simulink subsystem "FOC_Sub_StateMch"  (R2020b)
settings: Solver=VariableStepAuto  StartTime=0.0  StopTime=10.0  RelTol=1e-3
undefined symbols (not defined in the file or in its folder): innerPI, outerPI, Tctr
libraries: mcbcontrolslib x3
settings Model: Creator=k  LastModifiedBy=wangdi
settings OptimizationCC: DefaultParameterBehavior=Inlined  EnhancedBackFolding=on  PassReuseOutputArgsAs=Individual arguments  ZeroExternalMemoryAtStartup=off  ZeroInternalMemoryAtStartup=off  OptimizeBlockOrder=speed  DifferentSizesBufferReuse=on  OptimizationCustomize=off  EfficientTunableParamExpr=on
settings DebuggingCC: ParameterTunabilityLossMsg=error
settings SFSimCC: MATLABDynamicMemAlloc=off
settings RTWCC: Description=Embedded Coder  SystemTargetFile=ert.tlc  TemplateMakefile=ert_default_tmf
settings CodeAppCC: ForceParamTrailComments=on  IgnoreCustomStorageClasses=off  OperatorAnnotations=on  SimulinkDataObjDesc=on  SFDataObjDesc=on  InsertBlockDesc=on
settings ERTTargetCC: TargetLangStandard=C99 (ISO)  GenerateSampleERTMain=on  InlinedParameterPlacement=NonHierarchical  ERTCustomFileTemplate=example_file_process.tlc

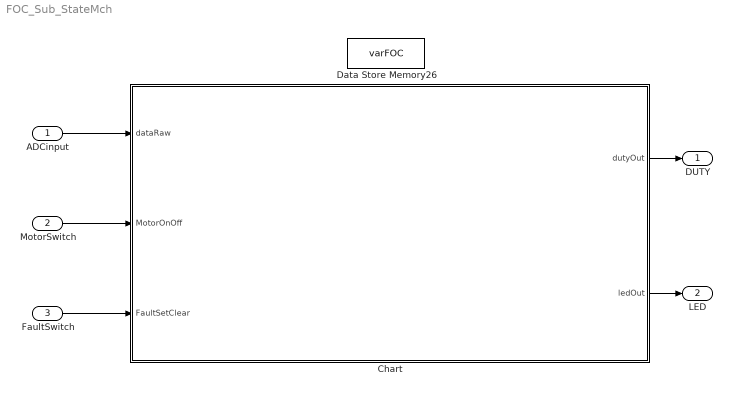
== system FOC_Sub_StateMch ==
  ADCinput : Inport  OutDataTypeStr=uint16  PortDimensions=5
  MotorSwitch : Inport  Port=2  OutDataTypeStr=boolean  PortDimensions=1
  FaultSwitch : Inport  Port=3  OutDataTypeStr=boolean  PortDimensions=1
  Chart : Stateflow chart  TreatAsAtomicUnit=on
  Data Store Memory26 : DataStoreMemory  DataStoreName=varFOC  ReadBeforeWriteMsg=warning  WriteAfterWriteMsg=warning  WriteAfterReadMsg=warning  ShowAdditionalParam=off  OutDataTypeStr=Bus: structFOC
  DUTY : Outport  PortDimensions=3
  LED : Outport  Port=2  PortDimensions=3
  wires:
  Chart/1(dutyOut) -> DUTY/1
  FaultSwitch/1 -> Chart/3(FaultSetClear)
  MotorSwitch/1 -> Chart/2(MotorOnOff)
  ADCinput/1 -> Chart/1(dataRaw)
  Chart/2(ledOut) -> LED/1

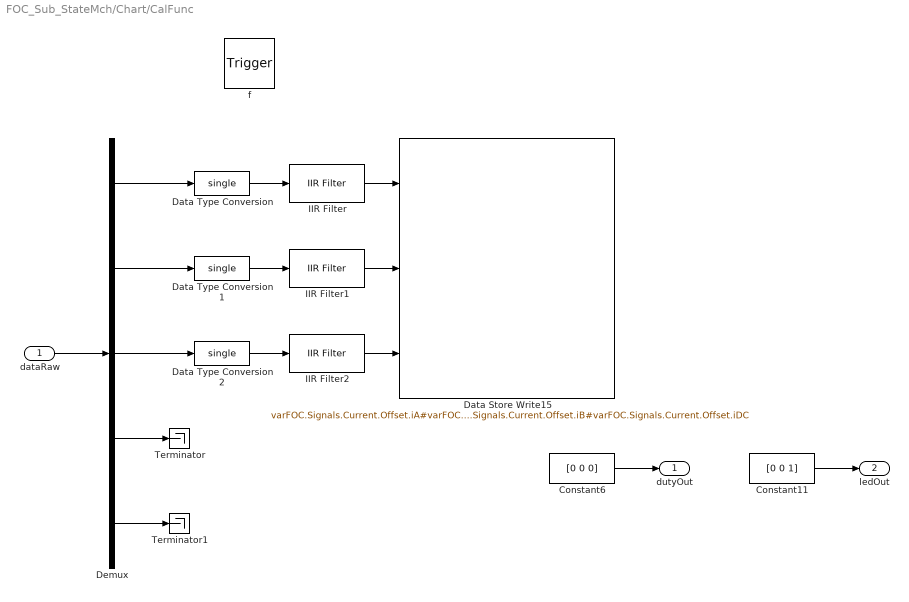
== system FOC_Sub_StateMch/Chart/CalFunc ==
  dataRaw : Inport  OutDataTypeStr=uint16  PortDimensions=5
  f : TriggerPort  TriggerType=function-call  VariantControl=(inherit)
      settings: CopyFcn=Stateflow.SLINSF.SimulinkMan.removeBlockPreDeleteFcn  PreDeleteFcn=Stateflow.SLINSF.SimulinkMan.unsafePredeleteFcn
  Constant11 : Constant  Value=[0 0 1]  OutDataTypeStr=boolean
  Constant6 : Constant  Value=[0 0 0]  OutDataTypeStr=single
  Data Store Write15 : DataStoreWrite  DataStoreName=varFOC  DataStoreElements=varFOC.Signals.Current.Offset.iA#varFOC.Signals.Current.Offset.iB#varFOC.Signals.Current.Offset.iDC
  Data Type Conversion : DataTypeConversion  OutDataTypeStr=single
  Data Type Conversion1 : DataTypeConversion  OutDataTypeStr=single
  Data Type Conversion2 : DataTypeConversion  OutDataTypeStr=single
  Demux : Demux  Outputs=5
  IIR Filter : mcbcontrolslib/IIR Filter  Filter_constant=0.001
      settings: SourceProductBaseCode=MT
  IIR Filter1 : mcbcontrolslib/IIR Filter  Filter_constant=0.001
      settings: SourceProductBaseCode=MT
  IIR Filter2 : mcbcontrolslib/IIR Filter  Filter_constant=0.001
      settings: SourceProductBaseCode=MT
  Terminator : Terminator
  Terminator1 : Terminator
  dutyOut : Outport  OutDataTypeStr=single
  ledOut : Outport  Port=2
  wires:
  IIR Filter2/1 -> Data Store Write15/3
  IIR Filter1/1 -> Data Store Write15/2
  Data Type Conversion2/1 -> IIR Filter2/1
  Demux/3 -> Data Type Conversion2/1
  Data Type Conversion1/1 -> IIR Filter1/1
  IIR Filter/1 -> Data Store Write15/1
  Demux/2 -> Data Type Conversion1/1
  Demux/1 -> Data Type Conversion/1
  Data Type Conversion/1 -> IIR Filter/1
  Demux/4 -> Terminator/1
  Demux/5 -> Terminator1/1
  dataRaw/1 -> Demux/1
  Constant6/1 -> dutyOut/1
  Constant11/1 -> ledOut/1

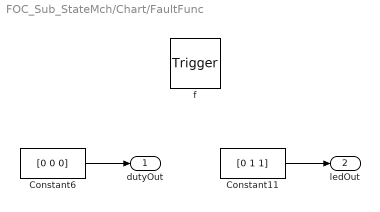
== system FOC_Sub_StateMch/Chart/FaultFunc ==
  f : TriggerPort  TriggerType=function-call  VariantControl=(inherit)
      settings: CopyFcn=Stateflow.SLINSF.SimulinkMan.removeBlockPreDeleteFcn  PreDeleteFcn=Stateflow.SLINSF.SimulinkMan.unsafePredeleteFcn
  Constant11 : Constant  Value=[0 1 1]  OutDataTypeStr=boolean
  Constant6 : Constant  Value=[0 0 0]  OutDataTypeStr=single
  dutyOut : Outport  OutDataTypeStr=single
  ledOut : Outport  Port=2
  wires:
  Constant6/1 -> dutyOut/1
  Constant11/1 -> ledOut/1

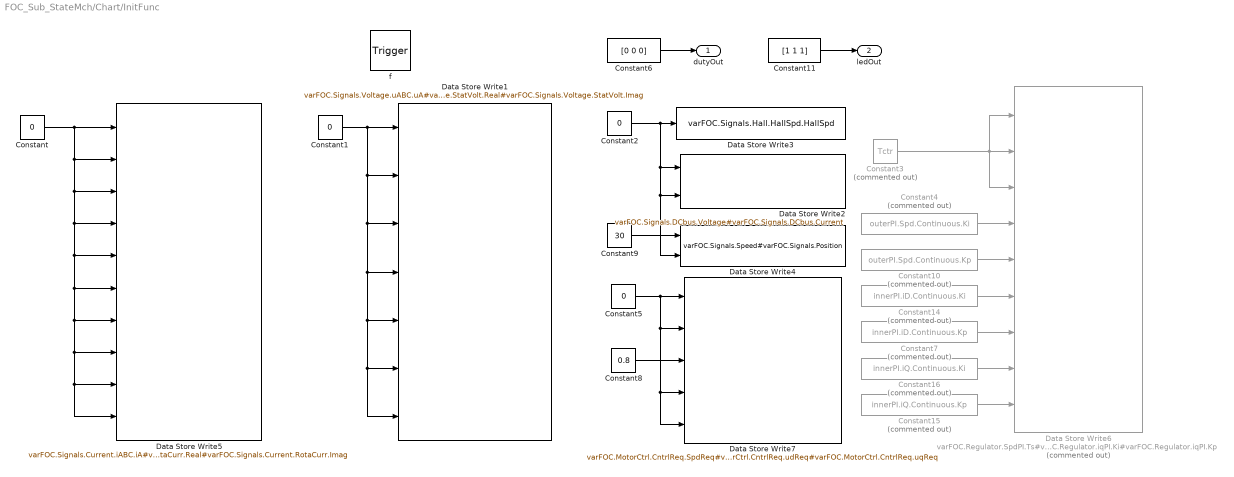
== system FOC_Sub_StateMch/Chart/InitFunc ==
  f : TriggerPort  TriggerType=function-call  VariantControl=(inherit)
      settings: CopyFcn=Stateflow.SLINSF.SimulinkMan.removeBlockPreDeleteFcn  PreDeleteFcn=Stateflow.SLINSF.SimulinkMan.unsafePredeleteFcn
  Constant{,1..2,5} (4 alike) : Constant  Value=0  OutDataTypeStr=single
  Constant10 : Constant  Commented=on  Value=outerPI.Spd.Continuous.Kp  OutDataTypeStr=single
  Constant11 : Constant  Value=[1 1 1]  OutDataTypeStr=boolean
  Constant14 : Constant  Commented=on  Value=innerPI.iD.Continuous.Ki  OutDataTypeStr=single
  Constant15 : Constant  Commented=on  Value=innerPI.iQ.Continuous.Kp  OutDataTypeStr=single
  Constant16 : Constant  Commented=on  Value=innerPI.iQ.Continuous.Ki  OutDataTypeStr=single
  Constant3 : Constant  Commented=on  Value=Tctr  OutDataTypeStr=single
  Constant4 : Constant  Commented=on  Value=outerPI.Spd.Continuous.Ki  OutDataTypeStr=single
  Constant6 : Constant  Value=[0 0 0]  OutDataTypeStr=single
  Constant7 : Constant  Commented=on  Value=innerPI.iD.Continuous.Kp  OutDataTypeStr=single
  Constant8 : Constant  Value=0.8  OutDataTypeStr=single
  Constant9 : Constant  Value=30  OutDataTypeStr=single
  Data Store Write1 : DataStoreWrite  DataStoreName=varFOC  DataStoreElements=varFOC.Signals.Voltage.uABC.uA#varFOC.Signals.Voltage.uABC.uB#varFOC.Signals.Voltage.uABC.uC#varFOC.Signals.Voltage.RotaVolt.Real#varFOC.Signals.Voltage.RotaVolt.Imag#varFOC.Signals.Voltage.StatVolt.Real#varFOC.Signals.Voltage.StatVolt.Imag
  Data Store Write2 : DataStoreWrite  DataStoreName=varFOC  DataStoreElements=varFOC.Signals.DCbus.Voltage#varFOC.Signals.DCbus.Current
  Data Store Write3 : DataStoreWrite  DataStoreName=varFOC  DataStoreElements=varFOC.Signals.Hall.HallSpd.HallSpd
  Data Store Write4 : DataStoreWrite  DataStoreName=varFOC  DataStoreElements=varFOC.Signals.Speed#varFOC.Signals.Position
  Data Store Write5 : DataStoreWrite  DataStoreName=varFOC  DataStoreElements=varFOC.Signals.Current.iABC.iA#varFOC.Signals.Current.iABC.iB#varFOC.Signals.Current.iABC.iC#varFOC.Signals.Current.Offset.iA#varFOC.Signals.Current.Offset.iB#varFOC.Signals.Current.Offset.iDC#varFOC.Signals.Current.StatCurr.Real#varFOC.Signals.Current.StatCurr.Imag#varFOC.Signals.Current.RotaCurr.Real#varFOC.Signals.Current.RotaCurr.Imag
  Data Store Write6 : DataStoreWrite  Commented=on  DataStoreName=varFOC  DataStoreElements=varFOC.Regulator.SpdPI.Ts#varFOC.Regulator.idPI.Ts#varFOC.Regulator.iqPI.Ts#varFOC.Regulator.SpdPI.Ki#varFOC.Regulator.SpdPI.Kp#varFOC.Regulator.idPI.Ki#varFOC.Regulator.idPI.Kp#varFOC.Regulator.iqPI.Ki#varFOC.Regulator.iqPI.Kp
  Data Store Write7 : DataStoreWrite  DataStoreName=varFOC  DataStoreElements=varFOC.MotorCtrl.CntrlReq.SpdReq#varFOC.MotorCtrl.CntrlReq.idReq#varFOC.MotorCtrl.CntrlReq.iqReq#varFOC.MotorCtrl.CntrlReq.udReq#varFOC.MotorCtrl.CntrlReq.uqReq
  dutyOut : Outport  OutDataTypeStr=single
  ledOut : Outport  Port=2
  wires:
  Constant4/1 -> Data Store Write6/4
  Constant10/1 -> Data Store Write6/5
  Constant16/1 -> Data Store Write6/8
  Constant/1 -> Data Store Write5/1, Data Store Write5/9, Data Store Write5/10, Data Store Write5/8, Data Store Write5/7, Data Store Write5/6, Data Store Write5/5, Data Store Write5/4, Data Store Write5/3, Data Store Write5/2
  Constant9/1 -> Data Store Write4/1
  Constant8/1 -> Data Store Write7/3
  Constant14/1 -> Data Store Write6/6
  Constant5/1 -> Data Store Write7/5, Data Store Write7/4, Data Store Write7/2, Data Store Write7/1
  Constant7/1 -> Data Store Write6/7
  Constant2/1 -> Data Store Write4/2, Data Store Write2/2, Data Store Write2/1, Data Store Write3/1
  Constant15/1 -> Data Store Write6/9
  Constant3/1 -> Data Store Write6/1, Data Store Write6/3, Data Store Write6/2
  Constant1/1 -> Data Store Write1/7, Data Store Write1/6, Data Store Write1/5, Data Store Write1/4, Data Store Write1/3, Data Store Write1/2, Data Store Write1/1
  Constant6/1 -> dutyOut/1
  Constant11/1 -> ledOut/1

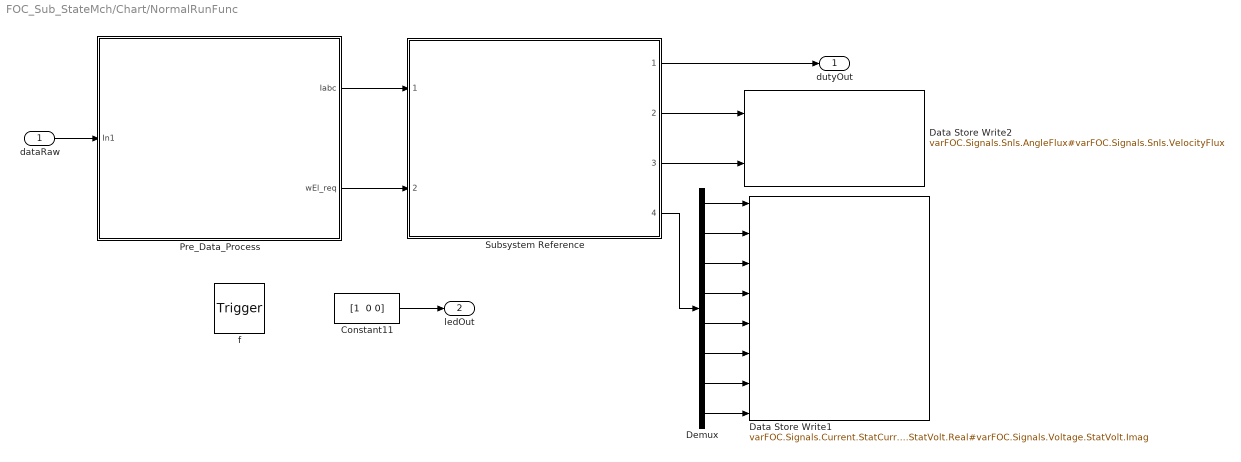
== system FOC_Sub_StateMch/Chart/NormalRunFunc ==
  dataRaw : Inport  OutDataTypeStr=uint16  PortDimensions=5
  f : TriggerPort  TriggerType=function-call  VariantControl=(inherit)
      settings: CopyFcn=Stateflow.SLINSF.SimulinkMan.removeBlockPreDeleteFcn  PreDeleteFcn=Stateflow.SLINSF.SimulinkMan.unsafePredeleteFcn
  Constant11 : Constant  Value="[1  0 0]"  OutDataTypeStr=boolean
  Data Store Write1 : DataStoreWrite  DataStoreName=varFOC  DataStoreElements=varFOC.Signals.Current.StatCurr.Real#varFOC.Signals.Current.StatCurr.Imag#varFOC.Signals.Current.RotaCurr.Real#varFOC.Signals.Current.RotaCurr.Imag#varFOC.Signals.Voltage.RotaVolt.Real#varFOC.Signals.Voltage.RotaVolt.Imag#varFOC.Signals.Voltage.StatVolt.Real#varFOC.Signals.Voltage.StatVolt.Imag
  Data Store Write2 : DataStoreWrite  DataStoreName=varFOC  DataStoreElements=varFOC.Signals.Snls.AngleFlux#varFOC.Signals.Snls.VelocityFlux
  Demux : Demux  Outputs=8
  Pre_Data_Process : Subsystem
  Subsystem Reference : Subsystem  ReferencedSubsystem=FOC_Sub_CoreAlgoithm
  dutyOut : Outport  OutDataTypeStr=single
  ledOut : Outport  Port=2
  wires:
  Pre_Data_Process/2(wEl_req) -> Subsystem Reference/2
  Pre_Data_Process/1(Iabc) -> Subsystem Reference/1
  Subsystem Reference/3 -> Data Store Write2/2
  Subsystem Reference/2 -> Data Store Write2/1
  Subsystem Reference/4 -> Demux/1
  Constant11/1 -> ledOut/1
  Subsystem Reference/1 -> dutyOut/1
  dataRaw/1 -> Pre_Data_Process/1(In1)
  Demux/1 -> Data Store Write1/1
  Demux/2 -> Data Store Write1/2
  Demux/3 -> Data Store Write1/3
  Demux/4 -> Data Store Write1/4
  Demux/5 -> Data Store Write1/5
  Demux/6 -> Data Store Write1/6
  Demux/7 -> Data Store Write1/7
  Demux/8 -> Data Store Write1/8

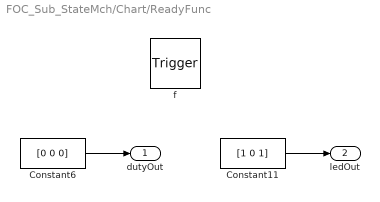
== system FOC_Sub_StateMch/Chart/ReadyFunc ==
  f : TriggerPort  TriggerType=function-call  VariantControl=(inherit)
      settings: CopyFcn=Stateflow.SLINSF.SimulinkMan.removeBlockPreDeleteFcn  PreDeleteFcn=Stateflow.SLINSF.SimulinkMan.unsafePredeleteFcn
  Constant11 : Constant  Value=[1 0 1]  OutDataTypeStr=boolean
  Constant6 : Constant  Value=[0 0 0]  OutDataTypeStr=single
  dutyOut : Outport  OutDataTypeStr=single
  ledOut : Outport  Port=2
  wires:
  Constant11/1 -> ledOut/1
  Constant6/1 -> dutyOut/1

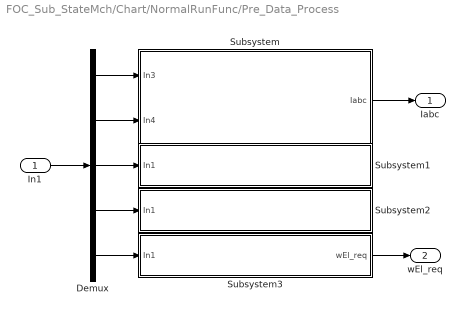
== system FOC_Sub_StateMch/Chart/NormalRunFunc/Pre_Data_Process ==
  In1 : Inport
  Demux : Demux  Outputs=5
  Subsystem : Subsystem
  Subsystem1 : Subsystem
  Subsystem2 : Subsystem
  Subsystem3 : Subsystem
  Iabc : Outport
  wEl_req : Outport  Port=2
  wires:
  Subsystem/1(Iabc) -> Iabc/1
  Demux/4 -> Subsystem2/1(In1)
  Demux/1 -> Subsystem/1(In3)
  Demux/5 -> Subsystem3/1(In1)
  Demux/3 -> Subsystem1/1(In1)
  Demux/2 -> Subsystem/2(In4)
  In1/1 -> Demux/1
  Subsystem3/1(wEl_req) -> wEl_req/1

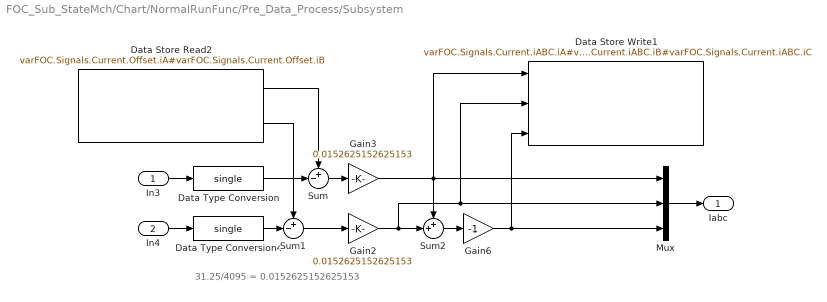
== system FOC_Sub_StateMch/Chart/NormalRunFunc/Pre_Data_Process/Subsystem ==
  note: 31.25/4095 = 0.0152625152625153
  In3 : Inport  OutDataTypeStr=uint16
  In4 : Inport  Port=2  OutDataTypeStr=uint16
  Data Store Read2 : DataStoreRead  DataStoreName=varFOC  DataStoreElements=varFOC.Signals.Current.Offset.iA#varFOC.Signals.Current.Offset.iB
  Data Store Write1 : DataStoreWrite  DataStoreName=varFOC  DataStoreElements=varFOC.Signals.Current.iABC.iA#varFOC.Signals.Current.iABC.iB#varFOC.Signals.Current.iABC.iC
  Data Type Conversion : DataTypeConversion  OutDataTypeStr=single
  Data Type Conversion4 : DataTypeConversion  OutDataTypeStr=single
  Gain2 : Gain  Gain=0.0152625152625153  OutDataTypeStr=single
  Gain3 : Gain  Gain=0.0152625152625153  OutDataTypeStr=single
  Gain6 : Gain  Gain=-1  OutDataTypeStr=single
  Mux : Mux  Inputs=3
  Sum : Sum  Inputs=+-|
  Sum1 : Sum  Inputs=+-|
  Sum2 : Sum  Inputs=++|
  Iabc : Outport
  wires:
  Mux/1 -> Iabc/1
  In4/1 -> Data Type Conversion4/1
  Data Type Conversion/1 -> Sum/2
  Gain3/1 -> Data Store Write1/1, Sum2/1, Mux/1
  Gain2/1 -> Data Store Write1/2, Mux/2, Sum2/2
  Sum2/1 -> Gain6/1
  Data Type Conversion4/1 -> Sum1/2
  Sum/1 -> Gain3/1
  Sum1/1 -> Gain2/1
  Data Store Read2/1 -> Sum/1
  In3/1 -> Data Type Conversion/1
  Data Store Read2/2 -> Sum1/1
  Gain6/1 -> Data Store Write1/3, Mux/3

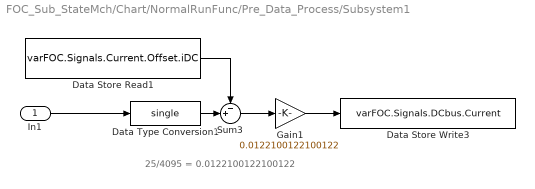
== system FOC_Sub_StateMch/Chart/NormalRunFunc/Pre_Data_Process/Subsystem1 ==
  note: 25/4095 = 0.0122100122100122
  In1 : Inport
  Data Store Read1 : DataStoreRead  DataStoreName=varFOC  DataStoreElements=varFOC.Signals.Current.Offset.iDC
  Data Store Write3 : DataStoreWrite  DataStoreName=varFOC  DataStoreElements=varFOC.Signals.DCbus.Current
  Data Type Conversion1 : DataTypeConversion  OutDataTypeStr=single
  Gain1 : Gain  Gain=0.0122100122100122  OutDataTypeStr=single
  Sum3 : Sum  Inputs=-+|
  wires:
  Data Store Read1/1 -> Sum3/1
  Sum3/1 -> Gain1/1
  Data Type Conversion1/1 -> Sum3/2
  Gain1/1 -> Data Store Write3/1
  In1/1 -> Data Type Conversion1/1

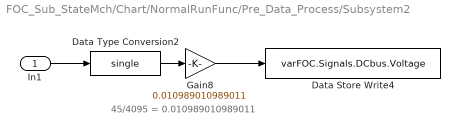
== system FOC_Sub_StateMch/Chart/NormalRunFunc/Pre_Data_Process/Subsystem2 ==
  note: 45/4095 = 0.010989010989011
  In1 : Inport
  Data Store Write4 : DataStoreWrite  DataStoreName=varFOC  DataStoreElements=varFOC.Signals.DCbus.Voltage
  Data Type Conversion2 : DataTypeConversion  OutDataTypeStr=single
  Gain8 : Gain  Gain=0.010989010989011  OutDataTypeStr=single
  wires:
  Data Type Conversion2/1 -> Gain8/1
  Gain8/1 -> Data Store Write4/1
  In1/1 -> Data Type Conversion2/1

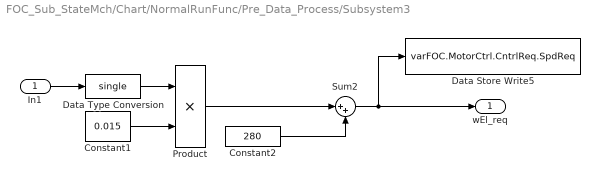
== system FOC_Sub_StateMch/Chart/NormalRunFunc/Pre_Data_Process/Subsystem3 ==
  In1 : Inport
  Constant1 : Constant  Value=0.015  OutDataTypeStr=single
  Constant2 : Constant  Value=280  OutDataTypeStr=single
  Data Store Write5 : DataStoreWrite  DataStoreName=varFOC  DataStoreElements=varFOC.MotorCtrl.CntrlReq.SpdReq
  Data Type Conversion : DataTypeConversion  OutDataTypeStr=single
  Product : Product
  Sum2 : Sum  Inputs=|++
  wEl_req : Outport
  wires:
  Constant2/1 -> Sum2/2
  Data Type Conversion/1 -> Product/1
  Sum2/1 -> Data Store Write5/1, wEl_req/1
  In1/1 -> Data Type Conversion/1
  Constant1/1 -> Product/2
  Product/1 -> Sum2/1

== stateflow chart FOC_Sub_StateMch/Chart ==
  state Run
    state Calibration
      en:CalCnt = 0;
      du:
      CalCnt = CalCnt + 1;
      [dutyOut, ledOut] = CalFunc(dataRaw);
    state NormalRun
      [dutyOut, ledOut] = NormalRunFunc(dataRaw);
    (default) -> Calibration
    Calibration -> NormalRun : [CalCnt > 10000]{CalCnt = 0;}
  state Initial
    [dutyOut, ledOut] = InitFunc();
    InitDone = true;
  state Ready
    [dutyOut, ledOut] = ReadyFunc();
  state Faults
    [dutyOut, ledOut] = FaultFunc();
  state [dutyOut,ledOut] = CalFunc(dataRaw) [function]
  state [dutyOut,ledOut] = InitFunc [function]
  state [dutyOut,ledOut] = FaultFunc [function]
  state [dutyOut,ledOut] = ReadyFunc [function]
  state [dutyOut,ledOut] = NormalRunFunc(dataRaw) [function]
  (default) -> Initial : {InitDone = false;}
  Run -> Initial [order 1] : [~MotorOnOff]{InitDone = false;}
  Initial -> Ready [order 1] : [InitDone]
  Ready -> Run [order 1] : [MotorOnOff]
  Faults -> Initial : [~FaultSetClear]{InitDone = false;}
  Initial -> Faults [order 2] : [FaultSetClear]
  Ready -> Faults [order 2] : [FaultSetClear]
  Run -> Faults [order 2] : [FaultSetClear]
  data: dataRaw function_input uint16 size=5; dutyOut function_output single; ledOut function_output; dutyOut function_output single; ledOut function_output; dutyOut function_output single; ledOut function_output; dutyOut function_output single; ledOut function_output; dutyOut function_output single; ledOut function_output; dataRaw function_input uint16 size=5; dataRaw input uint16 size=5; CalCnt local uint16 size=1; InitDone local boolean size=1; MotorOnOff input boolean size=1; FaultSetClear input boolean size=1; dutyOut output single size=3; ledOut output boolean size=3
